simulink model "gm_sampleModel1748_3_sub_sub"  (R2023a)
settings: Solver=VariableStepAuto  StartTime=0.0  StopTime=10.0  RelTol=1e-3
libraries: hdlsllib x6, simulink x1
settings Model: Creator=user1  LastModifiedBy=user1
settings OptimizationCC: BlockReduction=off  ConditionallyExecuteInputs=off
settings DebuggingCC: InheritedTsInSrcMsg=none

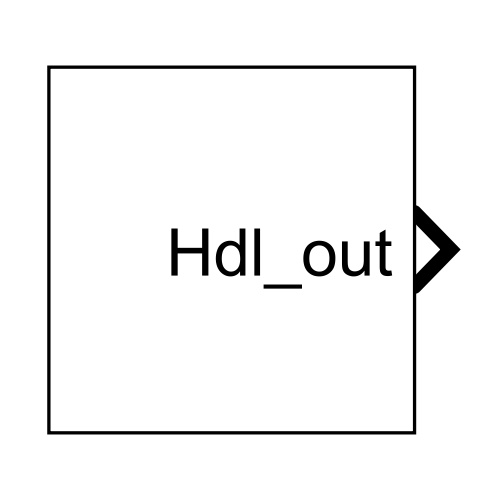
[thumbnail: Simulink's stored preview of the top-level diagram]
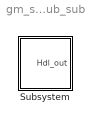
== system gm_sampleModel1748_3_sub_sub ==
  Subsystem : Subsystem

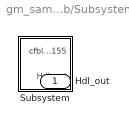
== system gm_sampleModel1748_3_sub_sub/Subsystem ==
  Subsystem : Subsystem
  Hdl_out : Outport  OutDataTypeStr=uint8

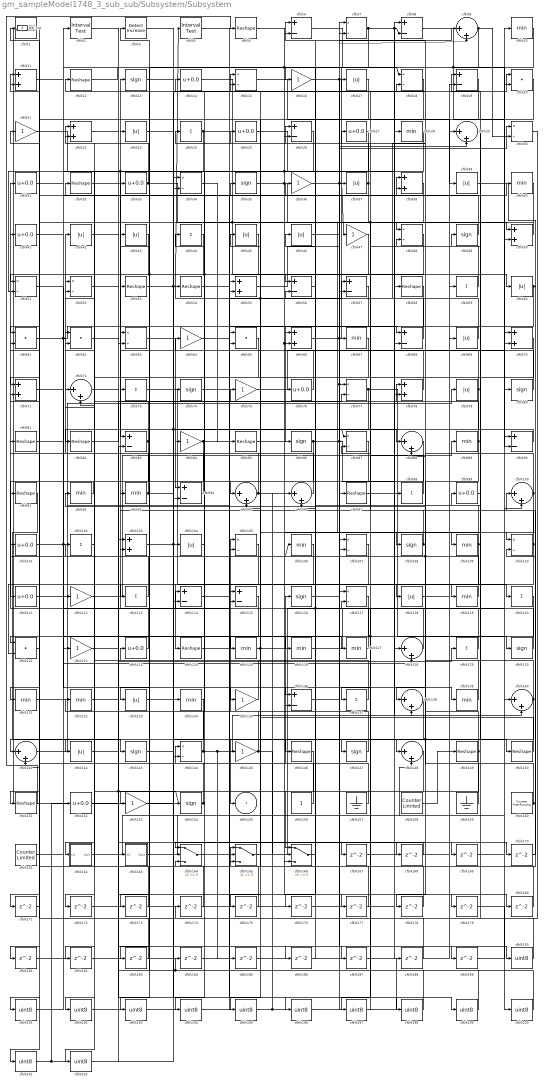
== system gm_sampleModel1748_3_sub_sub/Subsystem/Subsystem ==
  cfblk1 : hdlsllib/Logic and Bit Operations/Detect Fall Nonpositive  vinit=0  OutDataTypeStr=uint8
  cfblk{10,28,40,67,89,92..93,106,109,119,125..127,131..132,134,139} (17 alike) : MinMax  OutDataTypeStr=uint8
  cfblk{9,29,72,88,95..96,100,128,138,140..141,148} (12 alike) : Sum  Inputs=|++  OutDataTypeStr=uint8
  cfblk{14,25,27,31,33,41,76,99,101,111,123,152} (12 alike) : Bias  Bias=0.0  SaturateOnIntegerOverflow=off
  cfblk{24,44,59,73,98,102,113,120,129,137} (10 alike) : Sum  Inputs=+  OutDataTypeStr=uint8
  cfblk{11,22,38,50,55,66,70..71,78,103} (10 alike) : Sum  OutDataTypeStr=uint8
  cfblk{17,23,37,39,42..43,45..46,60,69,79,104,118,133,142} (15 alike) : Abs  OutDataTypeStr=uint8  SaturateOnIntegerOverflow=off
  cfblk{7,15,18,30,34,48,51..52,63,77,87,105,107,110,117,144} (16 alike) : Product  Inputs=*/  OutDataTypeStr=uint8  RndMeth=Zero  SaturateOnIntegerOverflow=on
  cfblk{13,35,49,74,80,86,108,116,130,143,147,154} (12 alike) : Signum
  cfblk{16,21,36,47,64,75,84,112,122,135,145,153} (12 alike) : Gain  OutDataTypeStr=uint8
  cfblk{6,8,19,26,56..57,68,83,90,94,114..115,136} (13 alike) : Sum  Inputs=+-  OutDataTypeStr=uint8
  cfblk{5,12,32,53..54,58,81..82,85,91,97,124,146,149..151} (16 alike) : Reshape
  cfblk{20,61..62,65,121} (5 alike) : DotProduct  OutDataTypeStr=uint8
  cfblk156 : Constant  OutDataTypeStr=uint8  SampleTime=-1
  cfblk157 : Ground
  cfblk158 : hdlsllib/Sources/Counter Limited  uplimit=7  tsamp=-1
  cfblk159 : Ground
  cfblk160 : hdlsllib/Sources/Counter Free-Running  NumBits=16  tsamp=-1
  cfblk161 : hdlsllib/Sources/Counter Limited  uplimit=7  tsamp=-1
  cfblk162 : Subsystem
      settings: LibrarySourceBlock=|
      | hdlsllib/Ports &
      | Subsystems/Subsystem
  cfblk163 : Subsystem
      settings: LibrarySourceBlock=|
      | hdlsllib/Ports &
      | Subsystems/Subsystem
  cfblk164 : Switch  OutDataTypeStr=uint8  SaturateOnIntegerOverflow=off  InputSameDT=off
  cfblk165 : Switch  OutDataTypeStr=uint8  SaturateOnIntegerOverflow=off  InputSameDT=off
  cfblk166 : Switch  OutDataTypeStr=uint8  SaturateOnIntegerOverflow=off  InputSameDT=off
  cfblk{167..189} (23 alike) : Delay  SampleTime=1
  cfblk{190..202} (13 alike) : DataTypeConversion  OutDataTypeStr=uint8  SaturateOnIntegerOverflow=off  RndMeth=Floor
  cfblk2 : hdlsllib/Logic and Bit Operations/Interval Test  IntervalClosedRight=on  uplimit=0.5  IntervalClosedLeft=on  lowlimit=-0.5  OutDataTypeStr=uint8
  cfblk3 : simulink/Logic and Bit Operations/Detect Increase  vinit=0.0  OutDataTypeStr=uint8
      settings: LibrarySourceBlock=|
      | hdlsllib/Logic and Bit
      | Operations/Detect
      | Increase
  cfblk4 : hdlsllib/Logic and Bit Operations/Interval Test  IntervalClosedRight=on  uplimit=0.5  IntervalClosedLeft=on  lowlimit=-0.5  OutDataTypeStr=uint8
  cfblk155 : Outport  OutDataTypeStr=uint8  VectorParamsAs1DForOutWhenUnconnected=off
  Hdl_out : Outport  Port=2  OutDataTypeStr=uint8
  wires:
  cfblk34/1 -> cfblk85/1
  cfblk156/1 -> cfblk116/1
  cfblk50/1 -> cfblk48/1
  cfblk73/1 -> cfblk119/1
  cfblk166/1 -> cfblk46/1
  cfblk123/1 -> cfblk13/1
  cfblk63/1 -> cfblk94/1
  cfblk12/1 -> cfblk67/1
  cfblk35/1 -> cfblk120/1, cfblk148/1
  cfblk153/1 -> cfblk74/1
  cfblk94/1 -> cfblk31/1
  cfblk24/1 -> cfblk90/2, cfblk51/2, cfblk83/1
  cfblk13/1 -> cfblk127/1, cfblk104/1
  cfblk36/1 -> cfblk189/1, cfblk47/1
  cfblk131/1 -> cfblk79/1
  cfblk18/1 -> cfblk95/1
  cfblk91/1 -> cfblk143/1
  cfblk93/1 -> cfblk15/1, cfblk42/1
  cfblk147/1 -> cfblk105/1
  cfblk68/1 -> cfblk6/1
  cfblk139/1 -> cfblk92/1
  cfblk125/1 -> cfblk175/1, cfblk28/1
  cfblk14/1 -> cfblk76/1, cfblk60/1
  cfblk77/1 -> cfblk145/1, cfblk130/1
  cfblk118/1 -> cfblk69/1
  cfblk112/1 -> cfblk89/1
  cfblk3/1 -> cfblk87/1, cfblk94/2
  cfblk129/1 -> cfblk41/1
  cfblk49/1 -> cfblk11/1
  cfblk138/1 -> cfblk155/1
  cfblk38/1 -> cfblk121/1
  cfblk79/1 -> cfblk114/2, cfblk26/1
  cfblk95/1 -> cfblk179/1, cfblk43/1
  cfblk134/1 -> cfblk201/1
  cfblk151/1 -> cfblk5/1
  cfblk9/1 -> cfblk173/1, cfblk30/2
  cfblk16/1 -> cfblk9/1, cfblk97/1
  cfblk19/1 -> cfblk61/1
  cfblk120/1 -> cfblk197/1, cfblk141/1
  cfblk105/1 -> cfblk151/1
  cfblk69/1 -> cfblk25/1, cfblk4/1
  cfblk137/1 -> cfblk23/1
  cfblk1/1 -> cfblk71/1
  cfblk37/1 -> cfblk15/2, cfblk73/1
  cfblk39/1 -> cfblk165/1
  cfblk158/1 -> cfblk149/1
  cfblk60/1 -> cfblk78/2, cfblk110/1
  cfblk141/1 -> cfblk34/1
  cfblk98/1 -> cfblk17/1
  cfblk84/1 -> cfblk147/1, cfblk111/1
  cfblk128/1 -> cfblk22/1, cfblk36/1
  cfblk140/1 -> cfblk35/1, cfblk106/1, cfblk168/1, cfblk167/1
  cfblk159/1 -> cfblk12/1
  cfblk102/1 -> cfblk32/1
  cfblk106/1 -> cfblk124/1
  cfblk144/1 -> cfblk132/1, cfblk185/1, cfblk140/2
  cfblk116/1 -> cfblk30/1, cfblk77/1
  cfblk76/1 -> cfblk3/1
  cfblk100/1 -> cfblk56/2, cfblk125/1
  cfblk117/1 -> cfblk195/1
  cfblk28/1 -> cfblk113/1, cfblk166/3, cfblk66/2
  cfblk104/1 -> cfblk14/1
  cfblk61/1 -> cfblk126/1, cfblk68/1
  cfblk31/1 -> cfblk37/1
  cfblk82/1 -> cfblk77/2
  cfblk87/1 -> cfblk131/1
  cfblk15/1 -> cfblk39/1
  cfblk165/1 -> cfblk80/1
  cfblk4/1 -> cfblk146/1
  cfblk46/1 -> cfblk88/1
  cfblk148/1 -> cfblk162/1(In1)
  cfblk133/1 -> cfblk150/1
  cfblk72/1 -> cfblk187/1, cfblk154/1
  cfblk86/1 -> cfblk115/2, cfblk138/2, cfblk107/1
  cfblk48/1 -> cfblk153/1
  cfblk55/1 -> cfblk7/1
  cfblk143/1 -> cfblk54/1
  cfblk110/1 -> cfblk87/2, cfblk138/1
  cfblk103/1 -> cfblk198/1
  cfblk145/1 -> cfblk166/2, cfblk44/1
  cfblk113/1 -> cfblk62/1
  cfblk92/1 -> cfblk91/1
  cfblk29/1 -> cfblk109/1
  cfblk163/1(Out1) -> cfblk148/2
  cfblk58/1 -> cfblk86/1
  cfblk21/1 -> cfblk165/2
  cfblk150/1 -> cfblk45/1
  cfblk81/1 -> cfblk122/1
  cfblk5/1 -> cfblk50/2, cfblk18/1
  cfblk51/1 -> cfblk112/1
  cfblk162/1(Out1) -> cfblk100/2
  cfblk32/1 -> cfblk33/1
  cfblk43/1 -> cfblk51/1
  cfblk108/1 -> cfblk93/1, cfblk88/2
  cfblk142/1 -> cfblk129/1
  cfblk25/1 -> cfblk98/1
  cfblk78/1 -> cfblk64/1
  cfblk89/1 -> cfblk178/1, cfblk62/2
  cfblk80/1 -> cfblk53/1
  cfblk164/1 -> cfblk55/1
  cfblk71/1 -> cfblk136/1
  cfblk115/1 -> cfblk164/1
  cfblk130/1 -> cfblk48/2
  cfblk127/1 -> cfblk81/1
  cfblk149/1 -> cfblk165/3, cfblk24/1
  cfblk83/1 -> cfblk52/2, cfblk142/1
  cfblk154/1 -> Hdl_out/1, cfblk144/1
  cfblk64/1 -> cfblk66/1
  cfblk111/1 -> cfblk128/2
  cfblk7/1 -> cfblk34/2, cfblk50/1, cfblk8/2
  cfblk17/1 -> cfblk26/2
  cfblk119/1 -> cfblk78/1, cfblk75/1
  cfblk33/1 -> cfblk22/2, cfblk90/1
  cfblk23/1 -> cfblk144/2
  cfblk97/1 -> cfblk20/1
  cfblk75/1 -> cfblk10/1
  cfblk126/1 -> cfblk59/1
  cfblk41/1 -> cfblk40/1
  cfblk45/1 -> cfblk63/2, cfblk84/1
  cfblk70/1 -> cfblk72/2
  cfblk157/1 -> cfblk21/1
  cfblk54/1 -> cfblk38/1
  cfblk10/1 -> cfblk56/1
  cfblk66/1 -> cfblk9/2, cfblk118/1
  cfblk96/1 -> cfblk52/1
  cfblk20/1 -> cfblk133/1
  cfblk122/1 -> cfblk135/1
  cfblk44/1 -> cfblk183/1, cfblk182/1
  cfblk22/1 -> cfblk163/1(In1)
  cfblk101/1 -> cfblk38/2, cfblk57/1
  cfblk40/1 -> cfblk96/2, cfblk137/1
  cfblk152/1 -> cfblk115/1
  cfblk135/1 -> cfblk102/1
  cfblk57/1 -> cfblk105/2
  cfblk160/1 -> cfblk110/2, cfblk101/1
  cfblk59/1 -> cfblk27/1
  cfblk85/1 -> cfblk108/1
  cfblk11/1 -> cfblk16/1
  cfblk136/1 -> cfblk29/2
  cfblk6/1 -> cfblk58/1
  cfblk146/1 -> cfblk166/1
  cfblk8/1 -> cfblk70/2, cfblk70/1
  cfblk90/1 -> cfblk82/1
  cfblk99/1 -> cfblk19/1
  cfblk161/1 -> cfblk114/1
  cfblk53/1 -> cfblk139/1, cfblk18/2
  cfblk109/1 -> cfblk121/2, cfblk63/1, cfblk49/1
  cfblk167/1 -> cfblk29/1
  cfblk168/1 -> cfblk164/2
  cfblk124/1 -> cfblk169/1
  cfblk169/1 -> cfblk140/1
  cfblk62/1 -> cfblk170/1
  cfblk170/1 -> cfblk100/1
  cfblk88/1 -> cfblk171/1
  cfblk171/1 -> cfblk11/2
  cfblk26/1 -> cfblk172/1
  cfblk172/1 -> cfblk107/2
  cfblk173/1 -> cfblk1/1
  cfblk30/1 -> cfblk174/1
  cfblk174/1 -> cfblk72/1
  cfblk175/1 -> cfblk164/3
  cfblk56/1 -> cfblk176/1
  cfblk176/1 -> cfblk8/1
  cfblk52/1 -> cfblk177/1
  cfblk177/1 -> cfblk6/2
  cfblk178/1 -> cfblk95/2
  cfblk74/1 -> cfblk180/1
  cfblk180/1 -> cfblk141/2
  cfblk121/1 -> cfblk181/1
  cfblk181/1 -> cfblk128/1
  cfblk182/1 -> cfblk55/2
  cfblk183/1 -> cfblk71/2
  cfblk184/1 -> cfblk19/2
  cfblk185/1 -> cfblk7/2
  cfblk132/1 -> cfblk186/1
  cfblk186/1 -> cfblk136/2
  cfblk187/1 -> cfblk68/2
  cfblk188/1 -> cfblk61/2
  cfblk189/1 -> cfblk20/2
  cfblk2/1 -> cfblk190/1
  cfblk190/1 -> cfblk99/1
  cfblk47/1 -> cfblk191/1
  cfblk191/1 -> cfblk2/1
  cfblk65/1 -> cfblk192/1
  cfblk192/1 -> cfblk188/1
  cfblk67/1 -> cfblk193/1
  cfblk193/1 -> cfblk65/1
  cfblk27/1 -> cfblk194/1
  cfblk194/1 -> cfblk65/2
  cfblk195/1 -> cfblk96/1, cfblk57/2
  cfblk114/1 -> cfblk196/1
  cfblk196/1 -> cfblk117/1
  cfblk197/1 -> cfblk117/2
  cfblk198/1 -> cfblk123/1, cfblk184/1
  cfblk42/1 -> cfblk199/1
  cfblk199/1 -> cfblk103/1
  cfblk179/1 -> cfblk200/1
  cfblk200/1 -> cfblk103/2
  cfblk201/1 -> cfblk152/1, cfblk83/2
  cfblk107/1 -> cfblk202/1
  cfblk202/1 -> cfblk134/1

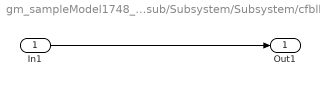
== system gm_sampleModel1748_3_sub_sub/Subsystem/Subsystem/cfblk162 ==
  In1 : Inport
  Out1 : Outport
  wires:
  In1/1 -> Out1/1

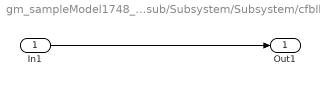
== system gm_sampleModel1748_3_sub_sub/Subsystem/Subsystem/cfblk163 ==
  In1 : Inport
  Out1 : Outport
  wires:
  In1/1 -> Out1/1
